simulink model "TVC3DOF"  (R2022b)
settings: Solver=VariableStepAuto  StartTime=0.0  StopTime=100  RelTol=1e-3
libraries: simulink x1, SignalEditorBlockLib x1
settings Model: Creator=alber  LastModifiedBy=alber

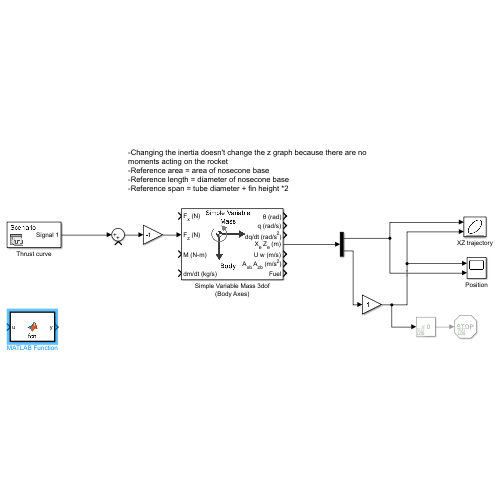
[thumbnail: Simulink's stored preview of the top-level diagram]
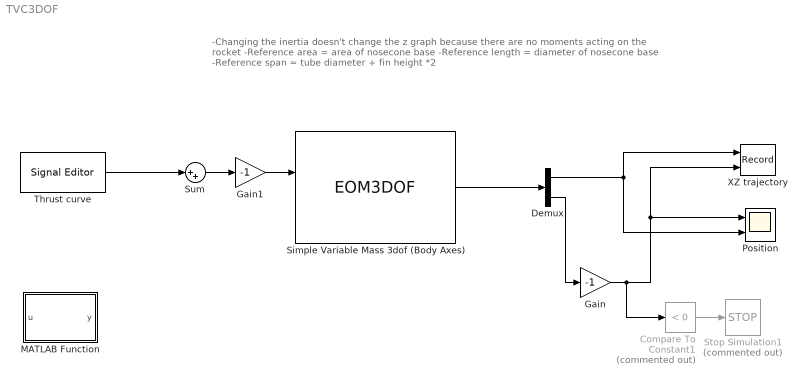
== system TVC3DOF ==
  note: -Changing the inertia doesn't change the z graph because there are no moments acting on the rocket
      | -Reference area = area of nosecone base
      | -Reference length = diameter of nosecone base
      | -Reference span = tube diameter + fin height *2
  Compare To Constant1 : simulink/Logic and Bit Operations/Compare To Constant  Commented=on  relop=<  const=0  OutDataTypeStr=boolean
  Demux : Demux  Outputs=2
  Gain : Gain  Gain=-1
  Gain1 : Gain  Gain=-1
  MATLAB Function : MATLAB Function  TreatAsAtomicUnit=on
  Position : Scope  NumInputPorts=2
  Simple Variable Mass 3dof (Body Axes) : EOM3DOF  mtype=Simple Variable  v_ini=0  mass=32.876  mass_e=19.568  mass_f=32.876  Iyy=0.095  Iyy_e=9.072  Iyy_f=12.043
  Stop Simulation1 : Stop  Commented=on
  Sum : Sum  Inputs=|++
  Thrust curve : SignalEditorBlockLib/Signal Editor  FileName=thrustcurve.mat  ActiveScenario=Scenario  ActiveSignal=Signal 1  IsBus=off  OutputBusObjectStr=Bus: BusObject  SampleTime=0  ZeroCross=off  OutputAfterFinalValue=Setting to zero  Unit=inherit  PreserveSignalName=on
  XZ trajectory : Record  FileSettingsInternal="{\"entries\":[{\"content\":{\"excelSettings\":{\"content\":{},\"type\":\"Streamout.ExcelSettings\"}},\"type\":\"Streamout.FileSettingStorage\",\"uuid\":\"a6013000-8eb7-432b-9878-c85ed96b091e\"}],\"packageUris\":[\"http://schema.mathworks.com/mf0/streamout_blocks/R2020a\"],\"version\":\"1.0\"}"  Layout=[1 1]  SignalsInternal="{\"entries\":[{\"content\":{\"signals\":[{\"content\":{\"blockPath\":[\"TVC3DOF/XZ trajectory\"],\"channel\":[],\"dimensions\":[1],\"domain\":\"TVC3DOF/XZ trajectory\",\"lineColor\":\"#a2142f\",\"plots\":[],\"port\":1,\"sid\":[],\"signalID\":8,\"signalName\":\"Demux:1\"},\"type\":\"RecordBlkView.Signal\",\"uuid\":\"cf19bc35-cd4f-47e3-bac3-14ab49063970\"},{\"content\":{\"blockPath\":[\"TVC3DOF/XZ trajectory\"],\"channel\":[],\"dimensions\":[1],\"domain\":\"TVC3DOF/XZ trajectory\",\"lineColor\":\"#139fff\",\"plots\":[],\"port\":2,\"sid\":[],\"signalID\":11,\"signalName\":\"Gain\"},\"type\":\"RecordBlkView.Signal\",\"uuid\":\"4291f71c-3f2f-4083-9d25-c714a911f470\"}]},\"type\":\"RecordBlkView.InputSignals\",\"uuid\":\"a980051e-fff9-4047-8af7-66f6e2fc4545\"}],\"packageUris\":[\"http://schema.mathworks.com/mf0/streamout_blocks/R2020a\"],\"version\":\"1.0\"}"  VisualizationBindings="{\"xyplotplugin\":{\"info\":[{\"series\":[],\"subplotID\":1}]}}"  CompatibilityTag=XY
  wires:
  Simple Variable Mass 3dof (Body Axes)/4 -> Demux/1
  Demux/1 -> Position/2, XZ trajectory/1
  Demux/2 -> Gain/1
  Gain/1 -> Compare To Constant1/1, XZ trajectory/2, Position/1
  Compare To Constant1/1 -> Stop Simulation1/1
  Gain1/1 -> Simple Variable Mass 3dof (Body Axes)/2
  Thrust curve/1 -> Sum/1
  Sum/1 -> Gain1/1

== matlab function TVC3DOF/MATLAB Function ==
  data: u input; y output
function y = fcn(u)

y = u;
